simulink model "pendolo"  (R2022a)
settings: Solver=ode45  StartTime=0.0  StopTime=15  MaxStep=0.01  RelTol=1e-3
values from neighbouring files (symbols this model uses):
  A = [0, 1; -g / l, -b / (m * l^2)]    [simulink_pendolo.m]
  b = 0    [simulink_pendolo.m]
  B = zeros(2, 1)    [simulink_pendolo.m]
  C = eye(2)    [simulink_pendolo.m]
  D = zeros(2, 1)    [simulink_pendolo.m]
  dot_th0 = 0    [simulink_pendolo.m]
  g = 9.81    [simulink_pendolo.m]
  l = 0.1    [simulink_pendolo.m]
  m = sin(th0 / 2)    [simulink_pendolo.m]
  th0 = 10 * deg2rad    (= 0.174532925199)    [simulink_pendolo.m]
  x0 = [th0; dot_th0]    [simulink_pendolo.m]
settings Model: Creator=loren  LastModifiedBy=loren
settings DataIOCC: ReturnWorkspaceOutputs=off

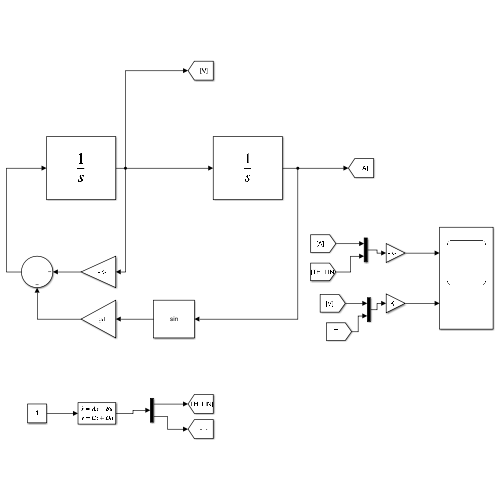
[thumbnail: Simulink's stored preview of the top-level diagram]
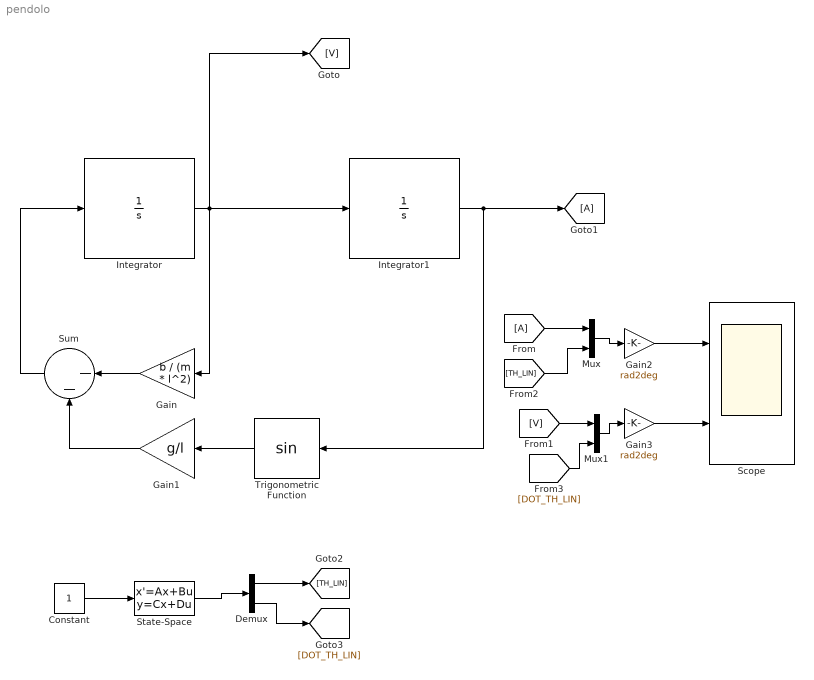
== system pendolo ==
  Constant : Constant
  Demux : Demux  Outputs=2
  From : From
  Gain : Gain  Gain=b / (m * l^2)
  Gain1 : Gain  Gain=g/l
  Gain2 : Gain  Gain=rad2deg
  Gain3 : Gain  Gain=rad2deg
  Goto1 : Goto
  Integrator : Integrator  InitialCondition=dot_th0
  Integrator1 : Integrator  InitialCondition=th0
  Mux : Mux  Inputs=2
  Mux1 : Mux  Inputs=2
  Scope : Scope  NumInputPorts=2
  State-Space : StateSpace  A=A  B=B  C=C  D=D  InitialCondition=x0
  Sum : Sum  Inputs=|--
  Trigonometric Function : Trigonometry
  wires:
  Integrator/1 -> [V], Gain/1, Integrator1/1
  Trigonometric Function/1 -> Gain1/1
  Integrator1/1 -> Goto1/1, Trigonometric Function/1
  Gain/1 -> Sum/1
  Gain1/1 -> Sum/2
  Sum/1 -> Integrator/1
  Gain2/1 -> Scope/1
  Gain3/1 -> Scope/2
  Constant/1 -> State-Space/1
  State-Space/1 -> Demux/1
  Demux/1 -> [TH_LIN]
  Demux/2 -> [DOT_TH_LIN]
  [V] -> Mux1/1
  [DOT_TH_LIN] -> Mux1/2
  Mux1/1 -> Gain3/1
  From/1 -> Mux/1
  [TH_LIN] -> Mux/2
  Mux/1 -> Gain2/1
